simulink model "sampleModel220"  (R2021b)
settings: Solver=VariableStepAuto  StartTime=0.0  StopTime=10.0  RelTol=1e-3
undefined symbols (not defined in the file or in its folder): Newton, Raphson
libraries: simulink x7, slpidlib x1
settings Model: Creator=user  LastModifiedBy=user

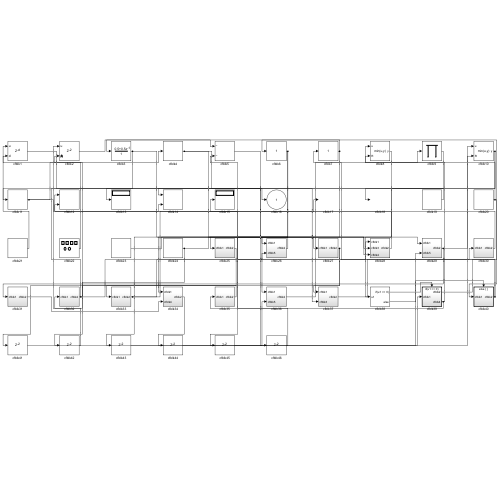
[thumbnail: Simulink's stored preview of the top-level diagram]
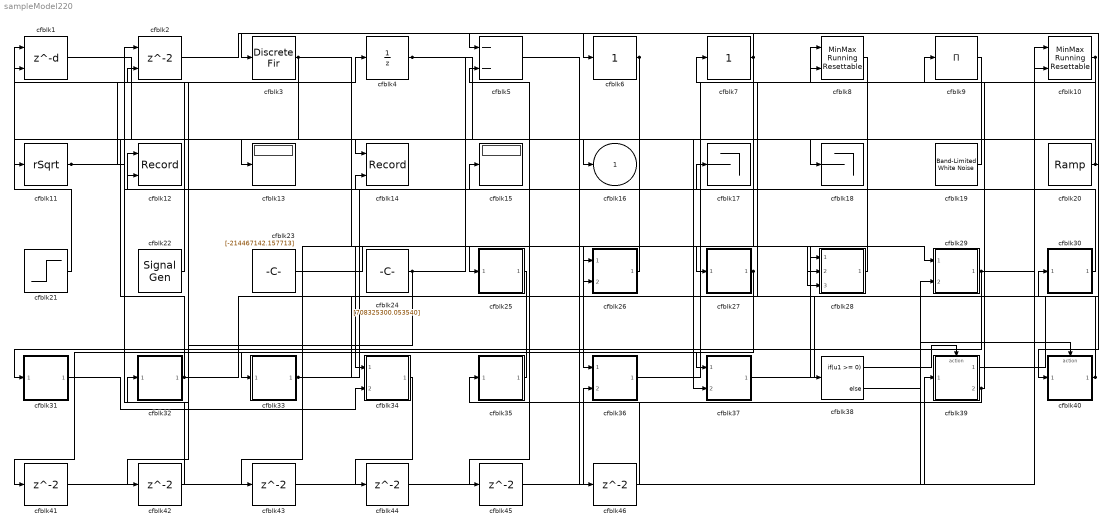
== system sampleModel220 ==
  cfblk1 : Delay  DelayLengthSource=Input port  SampleTime=1
      settings: InputPortMap=u0,p1
  cfblk10 : simulink/Math Operations/MinMax Running Resettable  Function=min  vinit=0.0
  cfblk11 : Sqrt  Operator=rSqrt  AlgorithmType=Newton-Raphson  SaturateOnIntegerOverflow=on
  cfblk12 : Record  FileSettingsInternal="{\"entries\":[{\"content\":{\"excelSettings\":{\"content\":{},\"type\":\"Streamout.ExcelSettings\"}},\"type\":\"Streamout.FileSettingStorage\",\"uuid\":\"505898ed-d4a3-4d30-8da6-12d5b21d2fb4\"}],\"packageUris\":[\"http://schema.mathworks.com/mf0/streamout_blocks/R2020a\"],\"version\":\"1.0\"}"  Layout=[1 1]  SignalsInternal="{\"entries\":[{\"content\":{\"signals\":[{\"content\":{\"blockPath\":[\"sampleModel220/cfblk12\"],\"channel\":[],\"dimensions\":[1],\"domain\":\"sampleModel220/cfblk12\",\"lineColor\":\"#a2142f\",\"plots\":[1],\"port\":1,\"sid\":[\"\"],\"signalID\":8544,\"signalName\":\"cfblk30\"},\"type\":\"RecordBlkView.Signal\",\"uuid\":\"e1a81a9f-4be3-4ea0-9128-7e2e516ad1fd\"},{\"content\":{\"blockPath\":[\"sampleModel220/cfblk12\"],\"channel\":[],\"dimensions\":[1],\"domain\":\"sampleModel220/cfblk12\",\"lineColor\":\"#139fff\",\"plots\":[1],\"port\":2,\"sid\":[\"\"],\"signalID\":8548,\"signalName\":\"cfblk28\"},\"type\":\"RecordBlkView.Signal\",\"uuid\":\"5418a6f3-f611-4ba8-824c-097e6ee0e848\"}]},\"type\":\"RecordBlkView.InputSignals\",\"uuid\":\"7c8a60f0-2ed5-44a6-9d5d-2e7e2406a068\"}],\"packageUris\":[\"http://schema.mathworks.com/mf0/streamout_blocks/R2020a\"],\"version\":\"1.0\"}"  VisualizationBindings="{\"xyplotplugin\":{\"info\":[{\"series\":[{\"bindingParametersList\":[{\"parameter\":\"X-Axis\",\"signalID\":8544,\"signalName\":\"cfblk30\"},{\"parameter\":\"Y-Axis\",\"signalID\":8548,\"signalName\":\"cfblk28\"}],\"seriesID\":16550}],\"subplotID\":1}]}}"  CompatibilityTag=XY
  cfblk13 : Display
  cfblk14 : Record  FileSettingsInternal="{\"entries\":[{\"content\":{\"excelSettings\":{\"content\":{},\"type\":\"Streamout.ExcelSettings\"}},\"type\":\"Streamout.FileSettingStorage\",\"uuid\":\"e3aca0db-b8d3-4546-a596-c9f2e1ed8f43\"}],\"packageUris\":[\"http://schema.mathworks.com/mf0/streamout_blocks/R2020a\"],\"version\":\"1.0\"}"  Layout=[1 1]  SignalsInternal="{\"entries\":[{\"content\":{\"signals\":[{\"content\":{\"blockPath\":[\"sampleModel220/cfblk14\"],\"channel\":[],\"dimensions\":[1],\"domain\":\"sampleModel220/cfblk14\",\"lineColor\":\"#a2142f\",\"plots\":[1],\"port\":1,\"sid\":[\"\"],\"signalID\":8552,\"signalName\":\"cfblk6\"},\"type\":\"RecordBlkView.Signal\",\"uuid\":\"0c1b1ec7-2b87-4732-9099-794a9beb898d\"},{\"content\":{\"blockPath\":[\"sampleModel220/cfblk14\"],\"channel\":[],\"dimensions\":[1,1],\"domain\":\"sampleModel220/cfblk14\",\"lineColor\":\"#139fff\",\"plots\":[1],\"port\":2,\"sid\":[\"\"],\"signalID\":8556,\"signalName\":\"cfblk11\"},\"type\":\"RecordBlkView.Signal\",\"uuid\":\"fc759081-9edc-4d6a-99ac-f6f69d52c412\"}]},\"type\":\"RecordBlkView.InputSignals\",\"uuid\":\"46ba40c3-e76c-4bd1-86ce-3226bd639f33\"}],\"packageUris\":[\"http://schema.mathworks.com/mf0/streamout_blocks/R2020a\"],\"version\":\"1.0\"}"  VisualizationBindings="{\"xyplotplugin\":{\"info\":[{\"series\":[{\"bindingParametersList\":[{\"parameter\":\"X-Axis\",\"signalID\":8552,\"signalName\":\"cfblk6\"},{\"parameter\":\"Y-Axis\",\"signalID\":8556,\"signalName\":\"cfblk11\"}],\"seriesID\":42241}],\"subplotID\":1}]}}"  CompatibilityTag=XY
  cfblk15 : Display
  cfblk17 : Terminator
  cfblk18 : Terminator
  cfblk19 : simulink/Sources/Band-Limited White Noise  Cov=[7884970699.678016]  Ts=0.1  seed=[4169388866.000000]
  cfblk2 : Delay  ShowEnablePort=on  SampleTime=1
      settings: InputPortMap=u0,e6
  cfblk20 : simulink/Sources/Ramp  slope=[5048.714924]  start=[38.839393]  InitialOutput=[657333.640343]
  cfblk21 : Step  Time=[43.000000]  Before=[104028622.435164]  After=[489802608.649629]  SampleTime=0
  cfblk22 : SignalGenerator  Amplitude=[831218374.420784]  Units=rad/sec
  cfblk23 : Constant  Value=[-214467142.157713]  SampleTime=1
  cfblk24 : Constant  Value=[708325300.053540]  SampleTime=1
  cfblk25 : Subsystem
  cfblk26 : Subsystem
  cfblk27 : Subsystem
  cfblk28 : Subsystem
  cfblk29 : Subsystem
  cfblk3 : DiscreteFir  SampleTime=1
  cfblk30 : Subsystem
  cfblk31 : Subsystem
  cfblk32 : Subsystem
  cfblk33 : Subsystem
  cfblk34 : Subsystem
  cfblk35 : Subsystem
  cfblk36 : Subsystem
  cfblk37 : Subsystem
  cfblk38 : If  IfExpression=u1 >= 0  SampleTime=1
  cfblk39 : Subsystem  TreatAsAtomicUnit=on
  cfblk4 : UnitDelay  HasFrameUpgradeWarning=on
  cfblk40 : Subsystem  TreatAsAtomicUnit=on
  cfblk{41..46} (6 alike) : Delay  SampleTime=1
  cfblk5 : Sum  Inputs=--
  cfblk6 : simulink/Math Operations/Slider Gain  gain=1  low=0  high=2
  cfblk7 : simulink/Math Operations/Slider Gain  gain=1  low=0  high=2
  cfblk8 : simulink/Math Operations/MinMax Running Resettable  Function=min  vinit=0.0
  cfblk9 : Product  Inputs=*
  cfblk16 : Outport
  wires:
  cfblk30/1(cfblk2) -> cfblk12/1
  cfblk35/1(cfblk2) -> cfblk33/1(cfblk1)
  cfblk32/1(cfblk2) -> cfblk16/1, cfblk28/1(cfblk1), cfblk2/2
  cfblk39/1(cfblk2) -> cfblk3/1
  cfblk24/1 -> cfblk32/1(cfblk1), cfblk28/2(cfblk3)
  cfblk10/1 -> cfblk36/1(cfblk1), cfblk11/1
  cfblk39/2(cfblk4) -> cfblk35/1(cfblk1), cfblk8/2
  cfblk19/1 -> cfblk18/1
  cfblk20/1 -> cfblk8/1, cfblk40/1(cfblk1)
  cfblk37/1(cfblk2) -> cfblk30/1(cfblk1)
  cfblk29/1(cfblk2) -> cfblk10/1, cfblk31/1(cfblk1)
  cfblk36/1(cfblk2) -> cfblk9/1
  cfblk11/1 -> cfblk4/1, cfblk14/2
  cfblk2/1 -> cfblk5/1
  cfblk21/1 -> cfblk1/1
  cfblk3/1 -> cfblk13/1, cfblk27/1(cfblk1)
  cfblk7/1 -> cfblk6/1, cfblk45/1
  cfblk5/1 -> cfblk29/1(cfblk1)
  cfblk33/1(cfblk2) -> cfblk17/1, cfblk26/2(cfblk5)
  cfblk27/1(cfblk2) -> cfblk37/1(cfblk1), cfblk41/1
  cfblk28/1(cfblk2) -> cfblk12/2
  cfblk4/1 -> cfblk28/3(cfblk4), cfblk46/1
  cfblk6/1 -> cfblk34/1(cfblk1), cfblk14/1
  cfblk26/1(cfblk2) -> cfblk25/1(cfblk1)
  cfblk31/1(cfblk2) -> cfblk34/2(cfblk4)
  cfblk9/1 -> cfblk38/1
  cfblk40/1(cfblk2) -> cfblk7/1, cfblk15/1
  cfblk22/1 -> cfblk1/2
  cfblk1/1 -> cfblk37/2(cfblk3)
  cfblk23/1 -> cfblk26/1(cfblk1)
  cfblk38/1 -> cfblk39/Action
  cfblk38/2 -> cfblk40/Action
  cfblk41/1 -> cfblk29/2(cfblk5)
  cfblk25/1(cfblk2) -> cfblk42/1
  cfblk42/1 -> cfblk2/1
  cfblk8/1 -> cfblk43/1
  cfblk43/1 -> cfblk39/1(cfblk1)
  cfblk34/1(cfblk2) -> cfblk44/1
  cfblk44/1 -> cfblk36/2(cfblk5)
  cfblk45/1 -> cfblk10/2
  cfblk46/1 -> cfblk5/2

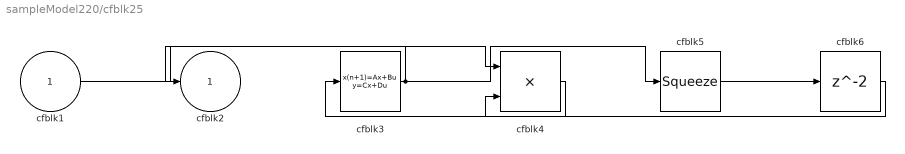
== system sampleModel220/cfblk25 ==
  cfblk1 : Inport
  cfblk3 : DiscreteStateSpace
  cfblk4 : Product
  cfblk5 : Squeeze
  cfblk6 : Delay  SampleTime=1
  cfblk2 : Outport
  wires:
  cfblk3/1 -> cfblk5/1, cfblk2/1
  cfblk1/1 -> cfblk4/1
  cfblk4/1 -> cfblk3/1
  cfblk5/1 -> cfblk6/1
  cfblk6/1 -> cfblk4/2

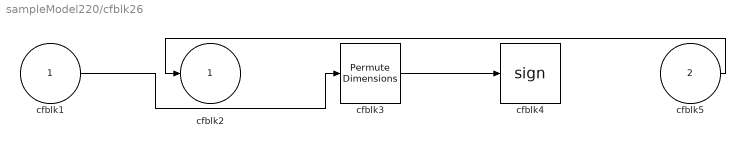
== system sampleModel220/cfblk26 ==
  cfblk1 : Inport
  cfblk5 : Inport  Port=2
  cfblk3 : PermuteDimensions
  cfblk4 : Signum
  cfblk2 : Outport
  wires:
  cfblk5/1 -> cfblk2/1
  cfblk1/1 -> cfblk3/1
  cfblk3/1 -> cfblk4/1

== system sampleModel220/cfblk27 ==
  cfblk1 : Inport
  cfblk3 : DiscreteFir  SampleTime=1
  cfblk2 : Outport
  wires:
  cfblk3/1 -> cfblk2/1
  cfblk1/1 -> cfblk3/1

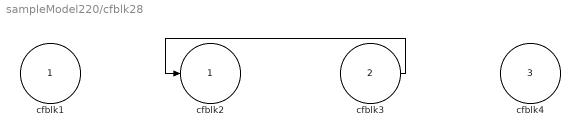
== system sampleModel220/cfblk28 ==
  cfblk1 : Inport
  cfblk3 : Inport  Port=2
  cfblk4 : Inport  Port=3
  cfblk2 : Outport
  wires:
  cfblk3/1 -> cfblk2/1

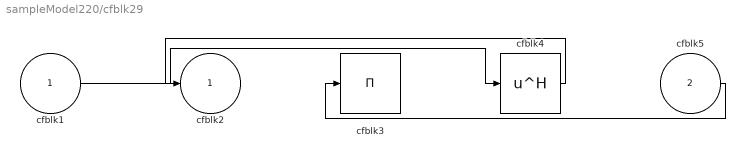
== system sampleModel220/cfblk29 ==
  cfblk1 : Inport
  cfblk5 : Inport  Port=2
  cfblk3 : Product  Inputs=*
  cfblk4 : Math  Operator=hermitian  SaturateOnIntegerOverflow=on
  cfblk2 : Outport
  wires:
  cfblk1/1 -> cfblk4/1
  cfblk5/1 -> cfblk3/1
  cfblk4/1 -> cfblk2/1

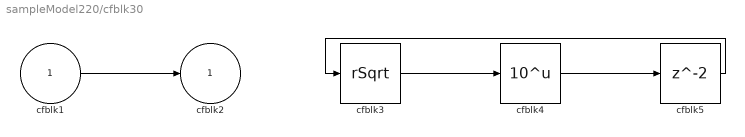
== system sampleModel220/cfblk30 ==
  cfblk1 : Inport
  cfblk3 : Sqrt  Operator=rSqrt  AlgorithmType=Newton-Raphson  SaturateOnIntegerOverflow=on
  cfblk4 : Math  Operator=10^u  SaturateOnIntegerOverflow=on
  cfblk5 : Delay  SampleTime=1
  cfblk2 : Outport
  wires:
  cfblk1/1 -> cfblk2/1
  cfblk3/1 -> cfblk4/1
  cfblk4/1 -> cfblk5/1
  cfblk5/1 -> cfblk3/1

== system sampleModel220/cfblk31 ==
  cfblk1 : Inport
  cfblk3 : Abs
  cfblk2 : Outport
  wires:
  cfblk1/1 -> cfblk3/1
  cfblk3/1 -> cfblk2/1

== system sampleModel220/cfblk32 ==
  cfblk1 : Inport
  cfblk3 : Trigonometry
  cfblk2 : Outport
  wires:
  cfblk1/1 -> cfblk2/1, cfblk3/1

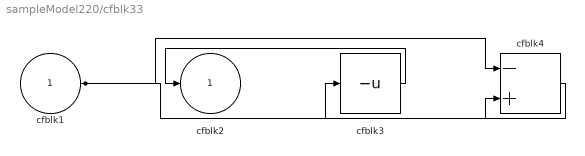
== system sampleModel220/cfblk33 ==
  cfblk1 : Inport
  cfblk3 : UnaryMinus
  cfblk4 : Sum  Inputs=-+
  cfblk2 : Outport
  wires:
  cfblk3/1 -> cfblk2/1
  cfblk1/1 -> cfblk4/1, cfblk4/2
  cfblk4/1 -> cfblk3/1

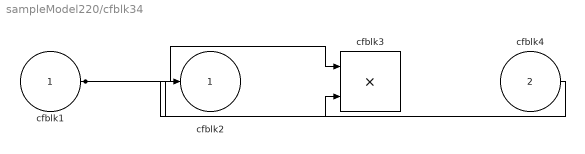
== system sampleModel220/cfblk34 ==
  cfblk1 : Inport
  cfblk4 : Inport  Port=2
  cfblk3 : Product
  cfblk2 : Outport
  wires:
  cfblk1/1 -> cfblk3/1, cfblk3/2
  cfblk4/1 -> cfblk2/1

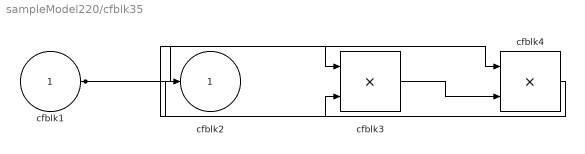
== system sampleModel220/cfblk35 ==
  cfblk1 : Inport
  cfblk3 : Product  Inputs=**
  cfblk4 : Product  Inputs=**
  cfblk2 : Outport
  wires:
  cfblk1/1 -> cfblk4/1, cfblk3/1, cfblk3/2
  cfblk4/1 -> cfblk2/1
  cfblk3/1 -> cfblk4/2

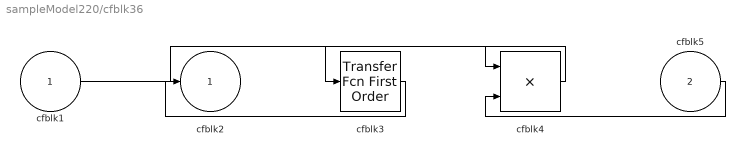
== system sampleModel220/cfblk36 ==
  cfblk1 : Inport
  cfblk5 : Inport  Port=2
  cfblk3 : simulink/Discrete/Transfer Fcn First Order  PoleZ=0.95  ICPrevOutput=0.0  DoSatur=off
  cfblk4 : Product  Inputs=**
  cfblk2 : Outport
  wires:
  cfblk1/1 -> cfblk4/1
  cfblk3/1 -> cfblk2/1
  cfblk5/1 -> cfblk4/2
  cfblk4/1 -> cfblk3/1

== system sampleModel220/cfblk37 ==
  cfblk1 : Inport
  cfblk3 : Inport  Port=2
  cfblk2 : Outport
  wires:
  cfblk3/1 -> cfblk2/1

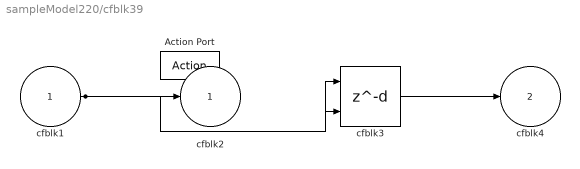
== system sampleModel220/cfblk39 ==
  cfblk1 : Inport
  Action Port : ActionPort  ActionPortLabel=if(u1 >= 0)
  cfblk3 : Delay  DelayLengthSource=Input port
      settings: InputPortMap=u0,p1
  cfblk2 : Outport
  cfblk4 : Outport  Port=2
  wires:
  cfblk1/1 -> cfblk2/1, cfblk3/1, cfblk3/2
  cfblk3/1 -> cfblk4/1

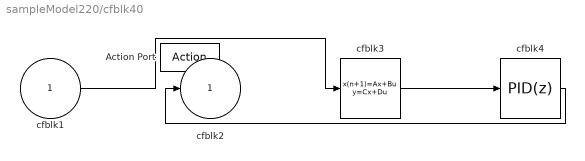
== system sampleModel220/cfblk40 ==
  cfblk1 : Inport
  Action Port : ActionPort  ActionPortLabel=else
  cfblk3 : DiscreteStateSpace  SampleTime=-1
  cfblk4 : slpidlib/PID Controller  Controller=PID  Form=Parallel  TimeDomain=Discrete-time  UseExternalTs=off  SampleTime=-1  IntegratorMethod=Forward Euler  FilterMethod=Forward Euler  ControllerParametersSource=internal  P=1  I=1  D=0  UseFilter=on  N=100  TunerSelectOption=Transfer Function Based (PID Tuner App)  InitialConditionSource=internal  InitialConditionForIntegrator=0  InitialConditionForFilter=0  DifferentiatorICPrevScaledInput=0  ExternalReset=none  TrackingMode=off  Kt=1  LimitOutput=off  SatLimitsSource=internal  UpperSaturationLimit=inf  LowerSaturationLimit=-inf  LinearizeAsGain=off  AntiWindupMode=none  Kb=1  POutMin=[]  POutMax=[]  IOutMin=[]  IOutMax=[]  DOutMin=[]  DOutMax=[]  NOutMin=[]  NOutMax=[]  SumOutMin=[]  SumOutMax=[]  SaturationOutMin=[]  SaturationOutMax=[]  PParamMin=[]  PParamMax=[]  IParamMin=[]  IParamMax=[]  DParamMin=[]  DParamMax=[]  NParamMin=[]  NParamMax=[]  KbParamMin=[]  KbParamMax=[]  KtParamMin=[]  KtParamMax=[]  KbOutMin=[]  KbOutMax=[]  KtOutMin=[]  KtOutMax=[]  IntegratorOutMin=[]  IntegratorOutMax=[]  FilterOutMin=[]  FilterOutMax=[]  SumI1OutMin=[]  SumI1OutMax=[]  SumI2OutMin=[]  SumI2OutMax=[]  SumI3OutMin=[]  SumI3OutMax=[]  SumI4OutMin=[]  SumI4OutMax=[]  SumDOutMin=[]  SumDOutMax=[]  DifferentiatorOutMin=[]  DifferentiatorOutMax=[]  FilterDiffOutCoefMin=[]  FilterDiffOutCoefMax=[]  ReciprocalOutMin=[]  ReciprocalOutMax=[]  SumDenOutMin=[]  SumDenOutMax=[]  SumNumOutMin=[]  SumNumOutMax=[]  DivideOutMin=[]  DivideOutMax=[]  UdiffTsProdOutMin=[]  UdiffTsProdOutMax=[]  NTsProdOutMin=[]  NTsProdOutMax=[]  UintegralTsProdOutMin=[]  UintegralTsProdOutMax=[]  UngainTsProdOutMin=[]  UngainTsProdOutMax=[]  IntegratorContinuousStateAttributes=''  IntegratorStateMustResolveToSignalObject=off  IntegratorRTWStateStorageClass=Auto  FilterContinuousStateAttributes=''  FilterStateMustResolveToSignalObject=off  FilterRTWStateStorageClass=Auto  ParallelPVariant=InternalParameters  IdealPVariant=Disabled  IVariant=InternalParameters  DVariant=InternalParameters  IntegratorVariant=Discrete  SatVariant=Disabled  AWVariant=Passthrough  PCopyVariant=Disabled  TRVariant=Disabled  FdbkBlocksVariant=Forward  IdealPFdbkVariant=Disabled  SatFdbkVariant=Disabled  DerivativeFilterVariant=ForwardEulerFilter  NVariant=InternalParameters  NCopyVariant=Disabled  FilterICVariant=InternalICsFilter  IntegratorICVariant=InternalICs  ExternalResetVariant=Disabled  TRSumVariant=Passthrough  SumFdbkVariant=Disabled  SumVariant=Sum_PID  TsampFilterVariant=InternalTs  TsampNgainVariant=Passthrough  TsampIntegralVariant=Passthrough  ExternalSaturationOutDataTypeStr=Inherit: Same as second input
  cfblk2 : Outport
  wires:
  cfblk4/1 -> cfblk2/1
  cfblk3/1 -> cfblk4/1
  cfblk1/1 -> cfblk3/1
